simulink library "MQM_lib"  (Simulink 7.5)
settings: Solver=ode45  StartTime=0.0  StopTime=10.0  RelTol=1e-3
values from neighbouring files (symbols this model uses):
  pMQM_Nm_MaxPreloadTrq_C = Simulink.Parameter    [MQM_par.m]
  pMQM_Nm_ShfTqLowrCrossHiThd_C = Simulink.Parameter    [MQM_par.m]
  pMQM_Nm_ShfTqLowrCrossThd_C = Simulink.Parameter    [MQM_par.m]
  pMQM_Nm_ShfTqUpprCrossHiThd_C = Simulink.Parameter    [MQM_par.m]
  pMQM_Nm_ShfTqUpprCrossThd_C = Simulink.Parameter    [MQM_par.m]
  pMQM_Nm_TqRecoverThd_C = Simulink.Parameter    [MQM_par.m]
  pMQM_r_ShfNearZeroFilterFac_C = Simulink.Parameter    [MQM_par.m]
  pMQM_r_ShfPastZeroFilterFac_C = Simulink.Parameter    [MQM_par.m]
  pMQM_r_ShfZeroCrsFilterFac_C = Simulink.Parameter    [MQM_par.m]
  pMQM_s_ShfTqZeroCrossTiout_C = Simulink.Parameter    [MQM_par.m]
undefined symbols (not defined in the file or in its folder): p_single_Minus_M, p_single_Plus_M, p_single_Zero_M
libraries: BaseOperationLib_Browser x48, simulink x1
settings Model: Creator=wuaibin  LastModifiedBy=wuaibin

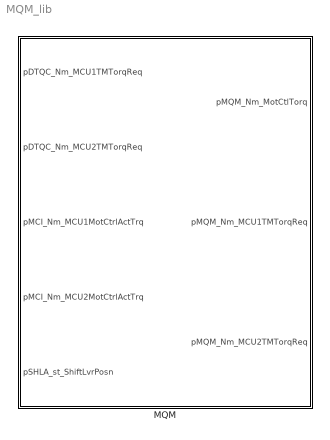
== system MQM_lib ==
  MQM : Subsystem  TreatAsAtomicUnit=on

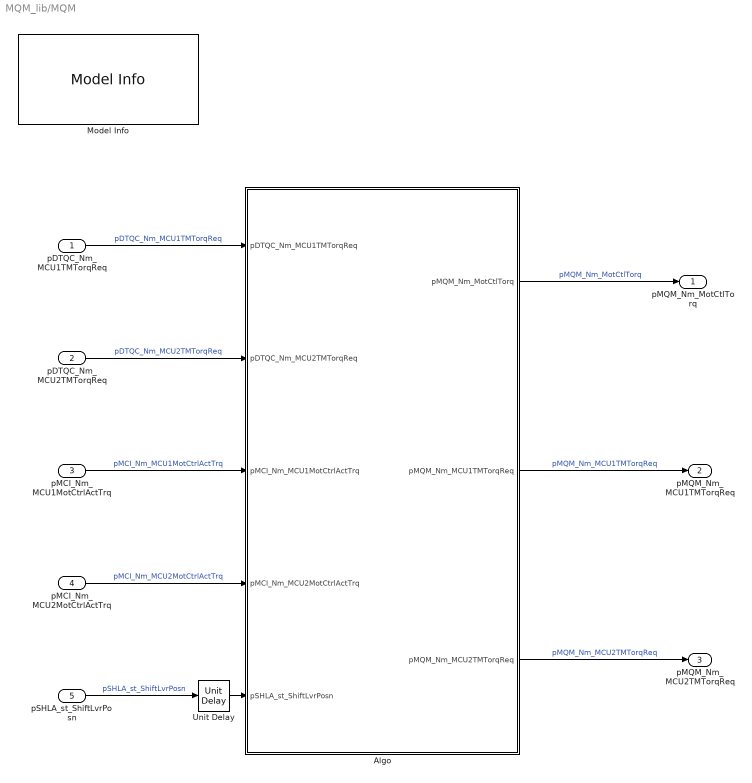
== system MQM_lib/MQM ==
  pDTQC_Nm_MCU1TMTorqReq : Inport
  pDTQC_Nm_MCU2TMTorqReq : Inport  Port=2
  pMCI_Nm_MCU1MotCtrlActTrq : Inport  Port=3
  pMCI_Nm_MCU2MotCtrlActTrq : Inport  Port=4
  pSHLA_st_ShiftLvrPosn : Inport  Port=5
  Algo : Subsystem
  Model Info : simulink/Model-Wide Utilities/Model Info  SystemSampleTime=-1  InitialBlockCM=None  BlockCM=None  Frame=on  DisplayStringWithTags=Model Info\nCreated: %<Created>\nCreator: %<Creator>  HorizontalTextAlignment=Center  LeftAlignmentValue=0.5  SourceBlockDiagram=untitled  TagMaxNumber=20
  Unit Delay : BaseOperationLib_Browser/Discrete Unchanged /Unit Delay  X0=0  SampleTime=-1
  pMQM_Nm_MotCtlTorq : Outport  OutDataType=fixdt(1, 16)  OutScaling=2^0
  pMQM_Nm_MCU1TMTorqReq : Outport  Port=2
  pMQM_Nm_MCU2TMTorqReq : Outport  Port=3
  wires:
  Unit Delay/1 -> Algo/5(pSHLA_st_ShiftLvrPosn)
  pDTQC_Nm_MCU1TMTorqReq/1 -> Algo/1(pDTQC_Nm_MCU1TMTorqReq)  "pDTQC_Nm_MCU1TMTorqReq"
  pDTQC_Nm_MCU2TMTorqReq/1 -> Algo/2(pDTQC_Nm_MCU2TMTorqReq)  "pDTQC_Nm_MCU2TMTorqReq"
  Algo/3(pMQM_Nm_MCU2TMTorqReq) -> pMQM_Nm_MCU2TMTorqReq/1  "pMQM_Nm_MCU2TMTorqReq"
  Algo/2(pMQM_Nm_MCU1TMTorqReq) -> pMQM_Nm_MCU1TMTorqReq/1  "pMQM_Nm_MCU1TMTorqReq"
  Algo/1(pMQM_Nm_MotCtlTorq) -> pMQM_Nm_MotCtlTorq/1  "pMQM_Nm_MotCtlTorq"
  pMCI_Nm_MCU1MotCtrlActTrq/1 -> Algo/3(pMCI_Nm_MCU1MotCtrlActTrq)  "pMCI_Nm_MCU1MotCtrlActTrq"
  pMCI_Nm_MCU2MotCtrlActTrq/1 -> Algo/4(pMCI_Nm_MCU2MotCtrlActTrq)  "pMCI_Nm_MCU2MotCtrlActTrq"
  pSHLA_st_ShiftLvrPosn/1 -> Unit Delay/1  "pSHLA_st_ShiftLvrPosn"

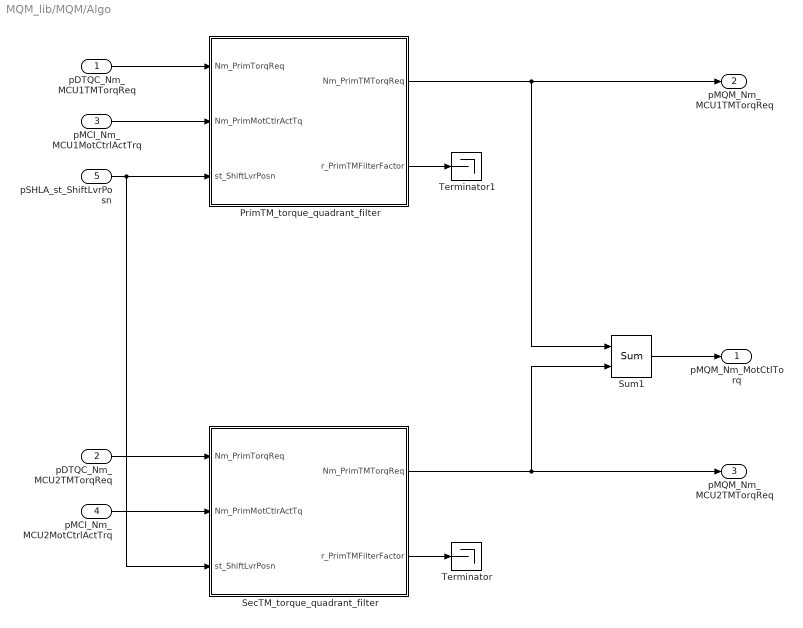
== system MQM_lib/MQM/Algo ==
  pDTQC_Nm_MCU1TMTorqReq : Inport
  pDTQC_Nm_MCU2TMTorqReq : Inport  Port=2
  pMCI_Nm_MCU1MotCtrlActTrq : Inport  Port=3
  pMCI_Nm_MCU2MotCtrlActTrq : Inport  Port=4
  pSHLA_st_ShiftLvrPosn : Inport  Port=5
  PrimTM_torque_quadrant_filter : Subsystem
  SecTM_torque_quadrant_filter : Subsystem
  Sum1 : BaseOperationLib_Browser/Math Operations Changed/Sum  Inputs=++  InputSameDT=on  OutMin=[]  OutMax=[]  OutDataType=fixdt(1, 16)  OutScaling=2^0  SaturateOnIntegerOverflow=on
  Terminator : Terminator
  Terminator1 : Terminator
  pMQM_Nm_MotCtlTorq : Outport  OutDataType=fixdt(1, 16)  OutScaling=2^0
  pMQM_Nm_MCU1TMTorqReq : Outport  Port=2
  pMQM_Nm_MCU2TMTorqReq : Outport  Port=3
  wires:
  pDTQC_Nm_MCU1TMTorqReq/1 -> PrimTM_torque_quadrant_filter/1(Nm_PrimTorqReq)
  pDTQC_Nm_MCU2TMTorqReq/1 -> SecTM_torque_quadrant_filter/1(Nm_PrimTorqReq)
  pMCI_Nm_MCU1MotCtrlActTrq/1 -> PrimTM_torque_quadrant_filter/2(Nm_PrimMotCtlrActTq)
  pSHLA_st_ShiftLvrPosn/1 -> SecTM_torque_quadrant_filter/3(st_ShiftLvrPosn), PrimTM_torque_quadrant_filter/3(st_ShiftLvrPosn)
  pMCI_Nm_MCU2MotCtrlActTrq/1 -> SecTM_torque_quadrant_filter/2(Nm_PrimMotCtlrActTq)
  SecTM_torque_quadrant_filter/2(r_PrimTMFilterFactor) -> Terminator/1
  PrimTM_torque_quadrant_filter/2(r_PrimTMFilterFactor) -> Terminator1/1
  PrimTM_torque_quadrant_filter/1(Nm_PrimTMTorqReq) -> pMQM_Nm_MCU1TMTorqReq/1, Sum1/1
  SecTM_torque_quadrant_filter/1(Nm_PrimTMTorqReq) -> pMQM_Nm_MCU2TMTorqReq/1, Sum1/2
  Sum1/1 -> pMQM_Nm_MotCtlTorq/1

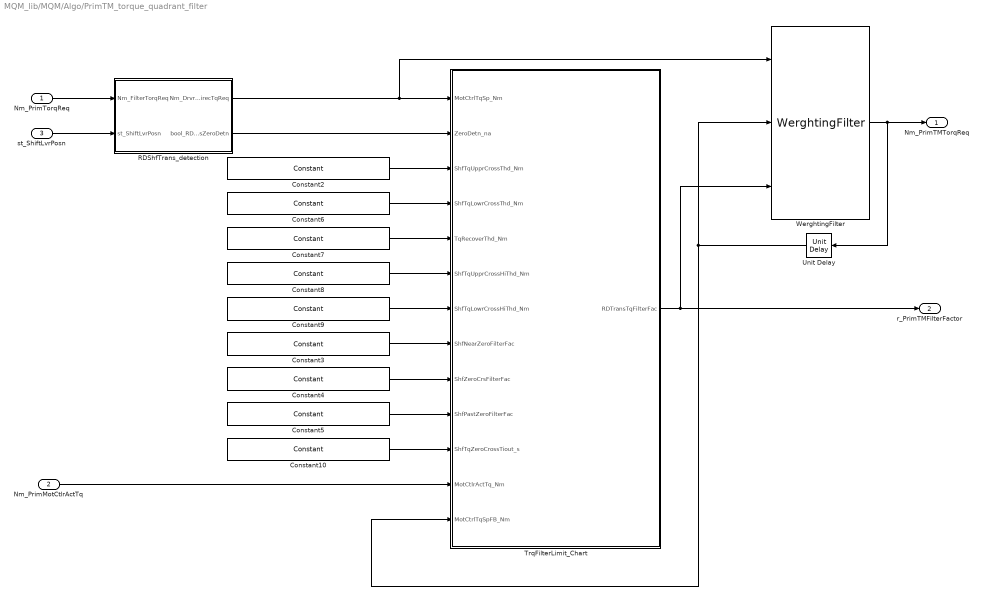
== system MQM_lib/MQM/Algo/PrimTM_torque_quadrant_filter ==
  Nm_PrimTorqReq : Inport
  Nm_PrimMotCtlrActTq : Inport  Port=2
  st_ShiftLvrPosn : Inport  Port=3
  Constant10 : BaseOperationLib_Browser/Sources&Sinks/Constant  Value=pMQM_s_ShfTqZeroCrossTiout_C  OutMin=[]  OutMax=[]  OutDataType=fixdt(1, 16)  ConRadixGroup=Use specified scaling  OutScaling=2^0  OutDataTypeStr=Inherit: Inherit from 'Constant value'
  Constant2 : BaseOperationLib_Browser/Sources&Sinks/Constant  Value=pMQM_Nm_ShfTqUpprCrossThd_C  OutMin=[]  OutMax=[]  OutDataType=fixdt(1, 16)  ConRadixGroup=Use specified scaling  OutScaling=2^0  OutDataTypeStr=Inherit: Inherit from 'Constant value'
  Constant3 : BaseOperationLib_Browser/Sources&Sinks/Constant  Value=pMQM_r_ShfNearZeroFilterFac_C  OutMin=[]  OutMax=[]  OutDataType=fixdt(1, 16)  ConRadixGroup=Use specified scaling  OutScaling=2^0  OutDataTypeStr=Inherit: Inherit from 'Constant value'
  Constant4 : BaseOperationLib_Browser/Sources&Sinks/Constant  Value=pMQM_r_ShfZeroCrsFilterFac_C  OutMin=[]  OutMax=[]  OutDataType=fixdt(1, 16)  ConRadixGroup=Use specified scaling  OutScaling=2^0  OutDataTypeStr=Inherit: Inherit from 'Constant value'
  Constant5 : BaseOperationLib_Browser/Sources&Sinks/Constant  Value=pMQM_r_ShfPastZeroFilterFac_C  OutMin=[]  OutMax=[]  OutDataType=fixdt(1, 16)  ConRadixGroup=Use specified scaling  OutScaling=2^0  OutDataTypeStr=Inherit: Inherit from 'Constant value'
  Constant6 : BaseOperationLib_Browser/Sources&Sinks/Constant  Value=pMQM_Nm_ShfTqLowrCrossThd_C  OutMin=[]  OutMax=[]  OutDataType=fixdt(1, 16)  ConRadixGroup=Use specified scaling  OutScaling=2^0  OutDataTypeStr=Inherit: Inherit from 'Constant value'
  Constant7 : BaseOperationLib_Browser/Sources&Sinks/Constant  Value=pMQM_Nm_TqRecoverThd_C  OutMin=[]  OutMax=[]  OutDataType=fixdt(1, 16)  ConRadixGroup=Use specified scaling  OutScaling=2^0  OutDataTypeStr=Inherit: Inherit from 'Constant value'
  Constant8 : BaseOperationLib_Browser/Sources&Sinks/Constant  Value=pMQM_Nm_ShfTqUpprCrossHiThd_C  OutMin=[]  OutMax=[]  OutDataType=fixdt(1, 16)  ConRadixGroup=Use specified scaling  OutScaling=2^0  OutDataTypeStr=Inherit: Inherit from 'Constant value'
  Constant9 : BaseOperationLib_Browser/Sources&Sinks/Constant  Value=pMQM_Nm_ShfTqLowrCrossHiThd_C  OutMin=[]  OutMax=[]  OutDataType=fixdt(1, 16)  ConRadixGroup=Use specified scaling  OutScaling=2^0  OutDataTypeStr=Inherit: Inherit from 'Constant value'
  RDShfTrans_detection : Subsystem
  TrqFilterLimit_Chart : Stateflow chart  TreatAsAtomicUnit=on
  Unit Delay : BaseOperationLib_Browser/Discrete Unchanged /Unit Delay  X0=0  SampleTime=-1
  WerghtingFilter : BaseOperationLib_Browser/Discontinuities Unchanged/WerghtingFilter  SystemSampleTime=-1
  Nm_PrimTMTorqReq : Outport
  r_PrimTMFilterFactor : Outport  Port=2
  wires:
  Constant10/1 -> TrqFilterLimit_Chart/11(ShfTqZeroCrossTiout_s)
  RDShfTrans_detection/1(Nm_DrvrDirecTqReq) -> WerghtingFilter/1, TrqFilterLimit_Chart/1(MotCtrlTqSp_Nm)
  Constant9/1 -> TrqFilterLimit_Chart/7(ShfTqLowrCrossHiThd_Nm)
  Constant8/1 -> TrqFilterLimit_Chart/6(ShfTqUpprCrossHiThd_Nm)
  Constant7/1 -> TrqFilterLimit_Chart/5(TqRecoverThd_Nm)
  Constant6/1 -> TrqFilterLimit_Chart/4(ShfTqLowrCrossThd_Nm)
  Constant2/1 -> TrqFilterLimit_Chart/3(ShfTqUpprCrossThd_Nm)
  st_ShiftLvrPosn/1 -> RDShfTrans_detection/2(st_ShiftLvrPosn)
  Constant5/1 -> TrqFilterLimit_Chart/10(ShfPastZeroFilterFac)
  Constant4/1 -> TrqFilterLimit_Chart/9(ShfZeroCrsFilterFac)
  Constant3/1 -> TrqFilterLimit_Chart/8(ShfNearZeroFilterFac)
  Nm_PrimMotCtlrActTq/1 -> TrqFilterLimit_Chart/12(MotCtlrActTq_Nm)
  Nm_PrimTorqReq/1 -> RDShfTrans_detection/1(Nm_FilterTorqReq)
  WerghtingFilter/1 -> Nm_PrimTMTorqReq/1, Unit Delay/1
  Unit Delay/1 -> TrqFilterLimit_Chart/13(MotCtrlTqSpFB_Nm), WerghtingFilter/2
  TrqFilterLimit_Chart/1(RDTransTqFilterFac) -> r_PrimTMFilterFactor/1, WerghtingFilter/3
  RDShfTrans_detection/2(bool_RDTransZeroDetn) -> TrqFilterLimit_Chart/2(ZeroDetn_na)

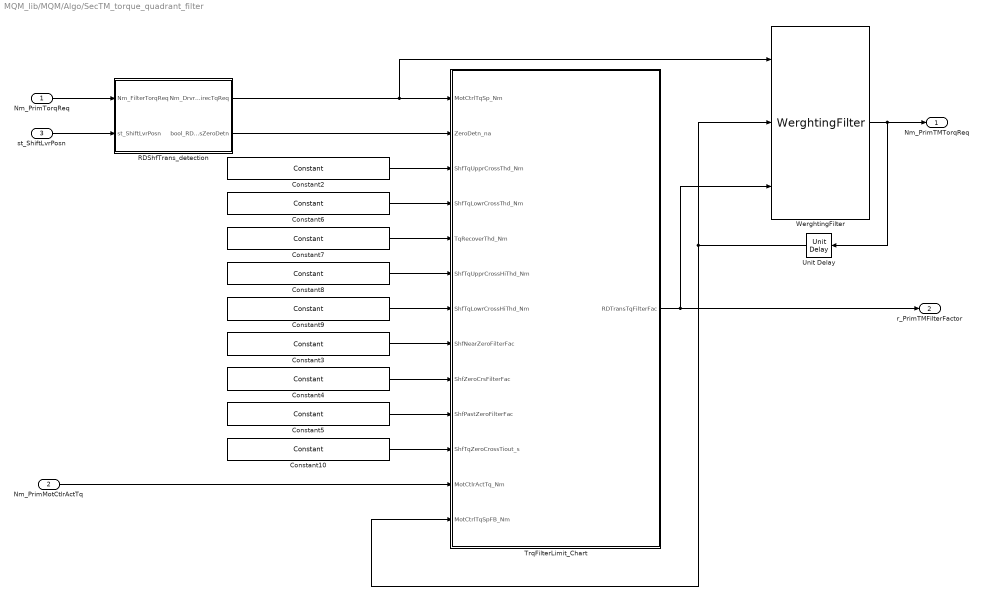
== system MQM_lib/MQM/Algo/SecTM_torque_quadrant_filter ==
  Nm_PrimTorqReq : Inport
  Nm_PrimMotCtlrActTq : Inport  Port=2
  st_ShiftLvrPosn : Inport  Port=3
  Constant10 : BaseOperationLib_Browser/Sources&Sinks/Constant  Value=pMQM_s_ShfTqZeroCrossTiout_C  OutMin=[]  OutMax=[]  OutDataType=fixdt(1, 16)  ConRadixGroup=Use specified scaling  OutScaling=2^0  OutDataTypeStr=Inherit: Inherit from 'Constant value'
  Constant2 : BaseOperationLib_Browser/Sources&Sinks/Constant  Value=pMQM_Nm_ShfTqUpprCrossThd_C  OutMin=[]  OutMax=[]  OutDataType=fixdt(1, 16)  ConRadixGroup=Use specified scaling  OutScaling=2^0  OutDataTypeStr=Inherit: Inherit from 'Constant value'
  Constant3 : BaseOperationLib_Browser/Sources&Sinks/Constant  Value=pMQM_r_ShfNearZeroFilterFac_C  OutMin=[]  OutMax=[]  OutDataType=fixdt(1, 16)  ConRadixGroup=Use specified scaling  OutScaling=2^0  OutDataTypeStr=Inherit: Inherit from 'Constant value'
  Constant4 : BaseOperationLib_Browser/Sources&Sinks/Constant  Value=pMQM_r_ShfZeroCrsFilterFac_C  OutMin=[]  OutMax=[]  OutDataType=fixdt(1, 16)  ConRadixGroup=Use specified scaling  OutScaling=2^0  OutDataTypeStr=Inherit: Inherit from 'Constant value'
  Constant5 : BaseOperationLib_Browser/Sources&Sinks/Constant  Value=pMQM_r_ShfPastZeroFilterFac_C  OutMin=[]  OutMax=[]  OutDataType=fixdt(1, 16)  ConRadixGroup=Use specified scaling  OutScaling=2^0  OutDataTypeStr=Inherit: Inherit from 'Constant value'
  Constant6 : BaseOperationLib_Browser/Sources&Sinks/Constant  Value=pMQM_Nm_ShfTqLowrCrossThd_C  OutMin=[]  OutMax=[]  OutDataType=fixdt(1, 16)  ConRadixGroup=Use specified scaling  OutScaling=2^0  OutDataTypeStr=Inherit: Inherit from 'Constant value'
  Constant7 : BaseOperationLib_Browser/Sources&Sinks/Constant  Value=pMQM_Nm_TqRecoverThd_C  OutMin=[]  OutMax=[]  OutDataType=fixdt(1, 16)  ConRadixGroup=Use specified scaling  OutScaling=2^0  OutDataTypeStr=Inherit: Inherit from 'Constant value'
  Constant8 : BaseOperationLib_Browser/Sources&Sinks/Constant  Value=pMQM_Nm_ShfTqUpprCrossHiThd_C  OutMin=[]  OutMax=[]  OutDataType=fixdt(1, 16)  ConRadixGroup=Use specified scaling  OutScaling=2^0  OutDataTypeStr=Inherit: Inherit from 'Constant value'
  Constant9 : BaseOperationLib_Browser/Sources&Sinks/Constant  Value=pMQM_Nm_ShfTqLowrCrossHiThd_C  OutMin=[]  OutMax=[]  OutDataType=fixdt(1, 16)  ConRadixGroup=Use specified scaling  OutScaling=2^0  OutDataTypeStr=Inherit: Inherit from 'Constant value'
  RDShfTrans_detection : Subsystem
  TrqFilterLimit_Chart : Stateflow chart  TreatAsAtomicUnit=on
  Unit Delay : BaseOperationLib_Browser/Discrete Unchanged /Unit Delay  X0=0  SampleTime=-1
  WerghtingFilter : BaseOperationLib_Browser/Discontinuities Unchanged/WerghtingFilter  SystemSampleTime=-1
  Nm_PrimTMTorqReq : Outport
  r_PrimTMFilterFactor : Outport  Port=2
  wires:
  RDShfTrans_detection/2(bool_RDTransZeroDetn) -> TrqFilterLimit_Chart/2(ZeroDetn_na)
  TrqFilterLimit_Chart/1(RDTransTqFilterFac) -> WerghtingFilter/3, r_PrimTMFilterFactor/1
  Unit Delay/1 -> WerghtingFilter/2, TrqFilterLimit_Chart/13(MotCtrlTqSpFB_Nm)
  WerghtingFilter/1 -> Unit Delay/1, Nm_PrimTMTorqReq/1
  Nm_PrimTorqReq/1 -> RDShfTrans_detection/1(Nm_FilterTorqReq)
  Nm_PrimMotCtlrActTq/1 -> TrqFilterLimit_Chart/12(MotCtlrActTq_Nm)
  Constant3/1 -> TrqFilterLimit_Chart/8(ShfNearZeroFilterFac)
  Constant4/1 -> TrqFilterLimit_Chart/9(ShfZeroCrsFilterFac)
  Constant5/1 -> TrqFilterLimit_Chart/10(ShfPastZeroFilterFac)
  st_ShiftLvrPosn/1 -> RDShfTrans_detection/2(st_ShiftLvrPosn)
  Constant2/1 -> TrqFilterLimit_Chart/3(ShfTqUpprCrossThd_Nm)
  Constant6/1 -> TrqFilterLimit_Chart/4(ShfTqLowrCrossThd_Nm)
  Constant7/1 -> TrqFilterLimit_Chart/5(TqRecoverThd_Nm)
  Constant8/1 -> TrqFilterLimit_Chart/6(ShfTqUpprCrossHiThd_Nm)
  Constant9/1 -> TrqFilterLimit_Chart/7(ShfTqLowrCrossHiThd_Nm)
  RDShfTrans_detection/1(Nm_DrvrDirecTqReq) -> TrqFilterLimit_Chart/1(MotCtrlTqSp_Nm), WerghtingFilter/1
  Constant10/1 -> TrqFilterLimit_Chart/11(ShfTqZeroCrossTiout_s)

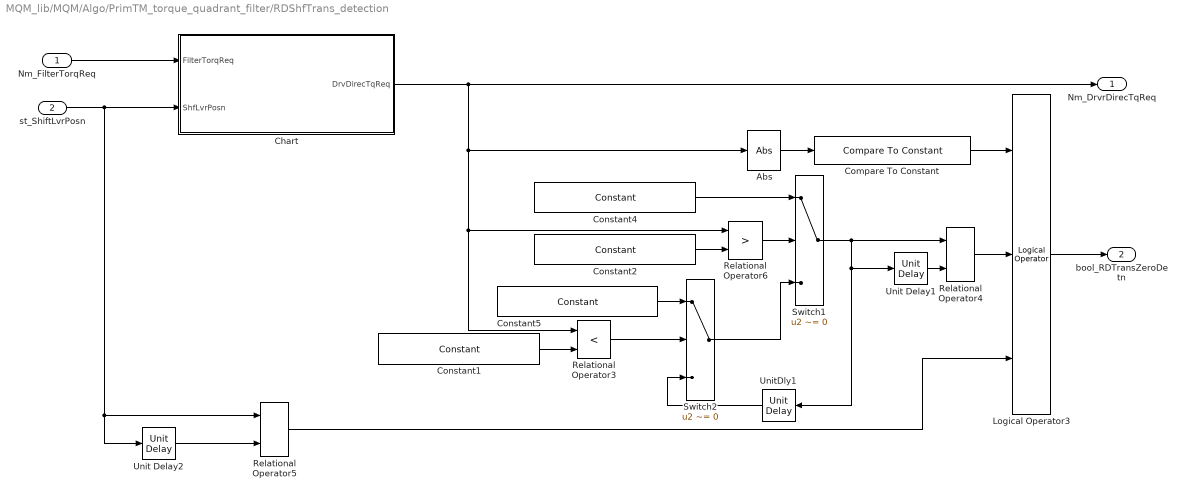
== system MQM_lib/MQM/Algo/PrimTM_torque_quadrant_filter/RDShfTrans_detection ==
  Nm_FilterTorqReq : Inport
  st_ShiftLvrPosn : Inport  Port=2
  Abs : BaseOperationLib_Browser/Math Operations Changed/Abs  OutMax=[]  OutDataType=fixdt(1, 16)  OutScaling=2^0  SaturateOnIntegerOverflow=on
  Chart : Stateflow chart  TreatAsAtomicUnit=on
  Compare To Constant : BaseOperationLib_Browser/Logic Operations Changed/Compare To Constant  SystemSampleTime=-1  relop=>=  const=pMQM_Nm_MaxPreloadTrq_C
  Constant1 : BaseOperationLib_Browser/Sources&Sinks/Constant  Value=p_single_Zero_M  OutMin=[]  OutMax=[]  OutDataType=fixdt(1, 16)  ConRadixGroup=Use specified scaling  OutScaling=2^0  OutDataTypeStr=Inherit: Inherit from 'Constant value'
  Constant2 : BaseOperationLib_Browser/Sources&Sinks/Constant  Value=p_single_Zero_M  OutMin=[]  OutMax=[]  OutDataType=fixdt(1, 16)  ConRadixGroup=Use specified scaling  OutScaling=2^0  OutDataTypeStr=Inherit: Inherit from 'Constant value'
  Constant4 : BaseOperationLib_Browser/Sources&Sinks/Constant  Value=p_single_Plus_M  OutMin=[]  OutMax=[]  OutDataType=fixdt(1, 16)  ConRadixGroup=Use specified scaling  OutScaling=2^0  OutDataTypeStr=Inherit: Inherit from 'Constant value'
  Constant5 : BaseOperationLib_Browser/Sources&Sinks/Constant  Value=p_single_Minus_M  OutMin=[]  OutMax=[]  OutDataType=fixdt(1, 16)  ConRadixGroup=Use specified scaling  OutScaling=2^0  OutDataTypeStr=Inherit: Inherit from 'Constant value'
  Logical Operator3 : BaseOperationLib_Browser/Logic Operations Changed/Logical Operator  Operator=AND  Inputs=3  AllPortsSameDT=off  OutDataTypeMode=boolean  LogicDataType=PDT_Bool  OutDataTypeStr=boolean
  Relational Operator3 : RelationalOperator  Operator=<  LogicOutDataTypeMode=Specify via dialog  LogicDataType=PDT_Bool  OutDataTypeStr=PDT_Bool  InputSameDT=on
      mask Display: patch([0 1 1 1 .75], [1 1 0 .75 1], [0 1 0]);
  Relational Operator4 : BaseOperationLib_Browser/Logic Operations Changed/Relational Operator  Operator=~=  InputSameDT=on  LogicOutDataTypeMode=Specify via dialog  LogicDataType=PDT_Bool  OutDataTypeStr=PDT_Bool
  Relational Operator5 : BaseOperationLib_Browser/Logic Operations Changed/Relational Operator  Operator=~=  InputSameDT=on  LogicOutDataTypeMode=Specify via dialog  LogicDataType=PDT_Bool  OutDataTypeStr=PDT_Bool
  Relational Operator6 : RelationalOperator  Operator=>  LogicOutDataTypeMode=Specify via dialog  LogicDataType=PDT_Bool  OutDataTypeStr=PDT_Bool  InputSameDT=on
      mask Display: patch([0 1 1 1 .75], [1 1 0 .75 1], [0 1 0]);
  Switch1 : Switch  Criteria=u2 ~= 0  Threshold=1  SaturateOnIntegerOverflow=on  InputSameDT=on
      mask Display: patch([0 1 1 1 .75], [1 1 0 .75 1], [0 1 0]);
  Switch2 : Switch  Criteria=u2 ~= 0  Threshold=1  SaturateOnIntegerOverflow=on  InputSameDT=on
      mask Display: patch([0 1 1 1 .75], [1 1 0 .75 1], [0 1 0]);
  Unit Delay1 : BaseOperationLib_Browser/Discrete Unchanged /Unit Delay  X0=0  SampleTime=-1
  Unit Delay2 : BaseOperationLib_Browser/Discrete Unchanged /Unit Delay  X0=0  SampleTime=-1
  UnitDly1 : BaseOperationLib_Browser/Discrete Unchanged /Unit Delay  X0=0  SampleTime=-1
  Nm_DrvrDirecTqReq : Outport
  bool_RDTransZeroDetn : Outport  Port=2
  wires:
  Relational Operator5/1 -> Logical Operator3/3
  Unit Delay2/1 -> Relational Operator5/2
  Constant5/1 -> Switch2/1
  Constant1/1 -> Relational Operator3/2
  Constant4/1 -> Switch1/1
  UnitDly1/1 -> Switch2/3
  Switch2/1 -> Switch1/3
  Relational Operator3/1 -> Switch2/2
  Switch1/1 -> Unit Delay1/1, UnitDly1/1, Relational Operator4/1
  Relational Operator6/1 -> Switch1/2
  Constant2/1 -> Relational Operator6/2
  st_ShiftLvrPosn/1 -> Unit Delay2/1, Relational Operator5/1, Chart/2(ShfLvrPosn)
  Nm_FilterTorqReq/1 -> Chart/1(FilterTorqReq)
  Chart/1(DrvDirecTqReq) -> Abs/1, Relational Operator3/1, Relational Operator6/1, Nm_DrvrDirecTqReq/1
  Logical Operator3/1 -> bool_RDTransZeroDetn/1
  Compare To Constant/1 -> Logical Operator3/1
  Abs/1 -> Compare To Constant/1
  Unit Delay1/1 -> Relational Operator4/2
  Relational Operator4/1 -> Logical Operator3/2

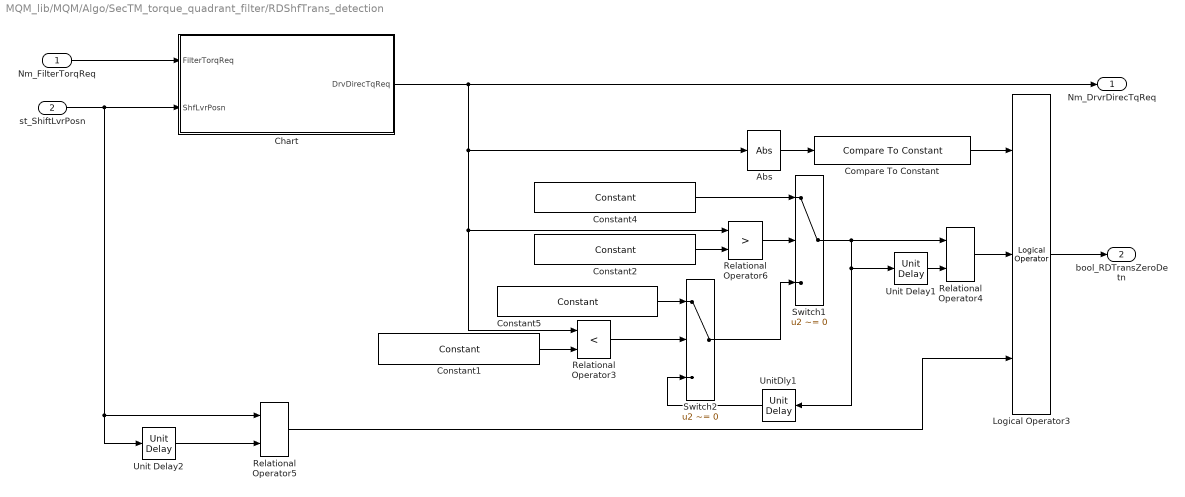
== system MQM_lib/MQM/Algo/SecTM_torque_quadrant_filter/RDShfTrans_detection ==
  Nm_FilterTorqReq : Inport
  st_ShiftLvrPosn : Inport  Port=2
  Abs : BaseOperationLib_Browser/Math Operations Changed/Abs  OutMax=[]  OutDataType=fixdt(1, 16)  OutScaling=2^0  SaturateOnIntegerOverflow=on
  Chart : Stateflow chart  TreatAsAtomicUnit=on
  Compare To Constant : BaseOperationLib_Browser/Logic Operations Changed/Compare To Constant  SystemSampleTime=-1  relop=>=  const=pMQM_Nm_MaxPreloadTrq_C
  Constant1 : BaseOperationLib_Browser/Sources&Sinks/Constant  Value=p_single_Zero_M  OutMin=[]  OutMax=[]  OutDataType=fixdt(1, 16)  ConRadixGroup=Use specified scaling  OutScaling=2^0  OutDataTypeStr=Inherit: Inherit from 'Constant value'
  Constant2 : BaseOperationLib_Browser/Sources&Sinks/Constant  Value=p_single_Zero_M  OutMin=[]  OutMax=[]  OutDataType=fixdt(1, 16)  ConRadixGroup=Use specified scaling  OutScaling=2^0  OutDataTypeStr=Inherit: Inherit from 'Constant value'
  Constant4 : BaseOperationLib_Browser/Sources&Sinks/Constant  Value=p_single_Plus_M  OutMin=[]  OutMax=[]  OutDataType=fixdt(1, 16)  ConRadixGroup=Use specified scaling  OutScaling=2^0  OutDataTypeStr=Inherit: Inherit from 'Constant value'
  Constant5 : BaseOperationLib_Browser/Sources&Sinks/Constant  Value=p_single_Minus_M  OutMin=[]  OutMax=[]  OutDataType=fixdt(1, 16)  ConRadixGroup=Use specified scaling  OutScaling=2^0  OutDataTypeStr=Inherit: Inherit from 'Constant value'
  Logical Operator3 : BaseOperationLib_Browser/Logic Operations Changed/Logical Operator  Operator=AND  Inputs=3  AllPortsSameDT=off  OutDataTypeMode=boolean  LogicDataType=PDT_Bool  OutDataTypeStr=boolean
  Relational Operator3 : RelationalOperator  Operator=<  LogicOutDataTypeMode=Specify via dialog  LogicDataType=PDT_Bool  OutDataTypeStr=PDT_Bool  InputSameDT=on
      mask Display: patch([0 1 1 1 .75], [1 1 0 .75 1], [0 1 0]);
  Relational Operator4 : BaseOperationLib_Browser/Logic Operations Changed/Relational Operator  Operator=~=  InputSameDT=on  LogicOutDataTypeMode=Specify via dialog  LogicDataType=PDT_Bool  OutDataTypeStr=PDT_Bool
  Relational Operator5 : BaseOperationLib_Browser/Logic Operations Changed/Relational Operator  Operator=~=  InputSameDT=on  LogicOutDataTypeMode=Specify via dialog  LogicDataType=PDT_Bool  OutDataTypeStr=PDT_Bool
  Relational Operator6 : RelationalOperator  Operator=>  LogicOutDataTypeMode=Specify via dialog  LogicDataType=PDT_Bool  OutDataTypeStr=PDT_Bool  InputSameDT=on
      mask Display: patch([0 1 1 1 .75], [1 1 0 .75 1], [0 1 0]);
  Switch1 : Switch  Criteria=u2 ~= 0  Threshold=1  SaturateOnIntegerOverflow=on  InputSameDT=on
      mask Display: patch([0 1 1 1 .75], [1 1 0 .75 1], [0 1 0]);
  Switch2 : Switch  Criteria=u2 ~= 0  Threshold=1  SaturateOnIntegerOverflow=on  InputSameDT=on
      mask Display: patch([0 1 1 1 .75], [1 1 0 .75 1], [0 1 0]);
  Unit Delay1 : BaseOperationLib_Browser/Discrete Unchanged /Unit Delay  X0=0  SampleTime=-1
  Unit Delay2 : BaseOperationLib_Browser/Discrete Unchanged /Unit Delay  X0=0  SampleTime=-1
  UnitDly1 : BaseOperationLib_Browser/Discrete Unchanged /Unit Delay  X0=0  SampleTime=-1
  Nm_DrvrDirecTqReq : Outport
  bool_RDTransZeroDetn : Outport  Port=2
  wires:
  Relational Operator4/1 -> Logical Operator3/2
  Unit Delay1/1 -> Relational Operator4/2
  Abs/1 -> Compare To Constant/1
  Compare To Constant/1 -> Logical Operator3/1
  Logical Operator3/1 -> bool_RDTransZeroDetn/1
  Chart/1(DrvDirecTqReq) -> Nm_DrvrDirecTqReq/1, Relational Operator6/1, Relational Operator3/1, Abs/1
  Nm_FilterTorqReq/1 -> Chart/1(FilterTorqReq)
  st_ShiftLvrPosn/1 -> Chart/2(ShfLvrPosn), Relational Operator5/1, Unit Delay2/1
  Constant2/1 -> Relational Operator6/2
  Relational Operator6/1 -> Switch1/2
  Switch1/1 -> Relational Operator4/1, UnitDly1/1, Unit Delay1/1
  Relational Operator3/1 -> Switch2/2
  Switch2/1 -> Switch1/3
  UnitDly1/1 -> Switch2/3
  Constant4/1 -> Switch1/1
  Constant1/1 -> Relational Operator3/2
  Constant5/1 -> Switch2/1
  Unit Delay2/1 -> Relational Operator5/2
  Relational Operator5/1 -> Logical Operator3/3

== stateflow chart MQM/Algo/SecTM_torque_quadrant_filter/RDShfTrans_detection/Chart ==
  state TQ_D
    en:
    DrvDirecTqReq=FilterTorqReq;
    du:
    DrvDirecTqReq=FilterTorqReq;
  state TQ_R
    en:
    DrvDirecTqReq=-FilterTorqReq;
    du:
    DrvDirecTqReq=-FilterTorqReq;
  TQ_D -> TQ_R : [ShfLvrPosn==ShiftLvrPosnTyp.SHL_R]
  TQ_R -> TQ_D : [ShfLvrPosn==ShiftLvrPosnTyp.SHL_D]
  (default) -> TQ_D
  data: FilterTorqReq input single; ShfLvrPosn input uint8; DrvDirecTqReq output single

== stateflow chart MQM/Algo/SecTM_torque_quadrant_filter/TrqFilterLimit_Chart ==
  state TorqueNoFilter
    en:
    RDTransTqFilterFac = 1;
    RisingZeroDetn_na=false;
    FallingZeroDetn_na=false;
    du:
    RDTransTqFilterFac = 1;
  state Shifting
    state ShiftZeroCrossingFilter
      en:
      RDTransTqFilterFac = ShfZeroCrsFilterFac;
      du:
      RDTransTqFilterFac = ShfZeroCrsFilterFac;
    state ShiftNearZeroFilter
      en:
      RDTransTqFilterFac = ShfNearZeroFilterFac;
      du:
      RDTransTqFilterFac = ShfNearZeroFilterFac;
    state ShiftPastZeroFilter
      en:
      RDTransTqFilterFac = ShfPastZeroFilterFac;
      du:
      RDTransTqFilterFac = ShfPastZeroFilterFac;
    ShiftNearZeroFilter -> ShiftZeroCrossingFilter : [(RisingZeroDetn_na&&MotCtlrActTq_Nm>= ShfTqUpprCrossThd_Nm)|| ...
        | (FallingZeroDetn_na&&MotCtlrActTq_Nm<=ShfTqLowrCrossThd_Nm)]
    ShiftZeroCrossingFilter -> ShiftPastZeroFilter : [(RisingZeroDetn_na&&MotCtlrActTq_Nm>= ShfTqUpprCrossHiThd_Nm)|| ...
        | (FallingZeroDetn_na&&MotCtlrActTq_Nm<=ShfTqLowrCrossHiThd_Nm)]
    (default) -> ShiftNearZeroFilter
  (default) -> TorqueNoFilter
  TorqueNoFilter -> Shifting [order 1] : [ZeroDetn_na&&(MotCtrlTqSp_Nm<0)]
      | {RisingZeroDetn_na=false;
      | FallingZeroDetn_na=true;}
  TorqueNoFilter -> Shifting [order 2] : [ZeroDetn_na&&(MotCtrlTqSp_Nm>0)]
      | {RisingZeroDetn_na=true;
      | FallingZeroDetn_na=false;}
  Shifting -> TorqueNoFilter : [(abs(MotCtrlTqSp_Nm-MotCtrlTqSpFB_Nm)<=TqRecoverThd_Nm)|| ...
      | (after(ShfTqZeroCrossTiout_s,sec))]
  data: MotCtrlTqSp_Nm input double; ZeroDetn_na input double; FallingZeroDetn_na local boolean; RDTransTqFilterFac output single; ShfTqUpprCrossThd_Nm input double; ShfTqLowrCrossThd_Nm input double; TqRecoverThd_Nm input double; ShfTqUpprCrossHiThd_Nm input double; ShfTqLowrCrossHiThd_Nm input double; ShfNearZeroFilterFac input double; ShfZeroCrsFilterFac input double; ShfPastZeroFilterFac input double; ShfTqZeroCrossTiout_s input double; MotCtlrActTq_Nm input double; MotCtrlTqSpFB_Nm input double; RisingZeroDetn_na local boolean

== stateflow chart MQM/Algo/PrimTM_torque_quadrant_filter/RDShfTrans_detection/Chart ==
  state TQ_D
    en:
    DrvDirecTqReq=FilterTorqReq;
    du:
    DrvDirecTqReq=FilterTorqReq;
  state TQ_R
    en:
    DrvDirecTqReq=-FilterTorqReq;
    du:
    DrvDirecTqReq=-FilterTorqReq;
  TQ_D -> TQ_R : [ShfLvrPosn==ShiftLvrPosnTyp.SHL_R]
  TQ_R -> TQ_D : [ShfLvrPosn==ShiftLvrPosnTyp.SHL_D]
  (default) -> TQ_D
  data: FilterTorqReq input single; ShfLvrPosn input uint8; DrvDirecTqReq output single

== stateflow chart MQM/Algo/PrimTM_torque_quadrant_filter/TrqFilterLimit_Chart ==
  state TorqueNoFilter
    en:
    RDTransTqFilterFac = 1;
    RisingZeroDetn_na=false;
    FallingZeroDetn_na=false;
    du:
    RDTransTqFilterFac = 1;
  state Shifting
    state ShiftZeroCrossingFilter
      en:
      RDTransTqFilterFac = ShfZeroCrsFilterFac;
      du:
      RDTransTqFilterFac = ShfZeroCrsFilterFac;
    state ShiftNearZeroFilter
      en:
      RDTransTqFilterFac = ShfNearZeroFilterFac;
      du:
      RDTransTqFilterFac = ShfNearZeroFilterFac;
    state ShiftPastZeroFilter
      en:
      RDTransTqFilterFac = ShfPastZeroFilterFac;
      du:
      RDTransTqFilterFac = ShfPastZeroFilterFac;
    ShiftNearZeroFilter -> ShiftZeroCrossingFilter : [(RisingZeroDetn_na&&MotCtlrActTq_Nm>= ShfTqUpprCrossThd_Nm)|| ...
        | (FallingZeroDetn_na&&MotCtlrActTq_Nm<=ShfTqLowrCrossThd_Nm)]
    ShiftZeroCrossingFilter -> ShiftPastZeroFilter : [(RisingZeroDetn_na&&MotCtlrActTq_Nm>= ShfTqUpprCrossHiThd_Nm)|| ...
        | (FallingZeroDetn_na&&MotCtlrActTq_Nm<=ShfTqLowrCrossHiThd_Nm)]
    (default) -> ShiftNearZeroFilter
  (default) -> TorqueNoFilter
  TorqueNoFilter -> Shifting [order 1] : [ZeroDetn_na&&(MotCtrlTqSp_Nm<0)]
      | {RisingZeroDetn_na=false;
      | FallingZeroDetn_na=true;}
  TorqueNoFilter -> Shifting [order 2] : [ZeroDetn_na&&(MotCtrlTqSp_Nm>0)]
      | {RisingZeroDetn_na=true;
      | FallingZeroDetn_na=false;}
  Shifting -> TorqueNoFilter : [(abs(MotCtrlTqSp_Nm-MotCtrlTqSpFB_Nm)<=TqRecoverThd_Nm)|| ...
      | (after(ShfTqZeroCrossTiout_s,sec))]
  data: MotCtrlTqSp_Nm input double; ZeroDetn_na input double; FallingZeroDetn_na local boolean; RDTransTqFilterFac output single; ShfTqUpprCrossThd_Nm input double; ShfTqLowrCrossThd_Nm input double; TqRecoverThd_Nm input double; ShfTqUpprCrossHiThd_Nm input double; ShfTqLowrCrossHiThd_Nm input double; ShfNearZeroFilterFac input double; ShfZeroCrsFilterFac input double; ShfPastZeroFilterFac input double; ShfTqZeroCrossTiout_s input double; MotCtlrActTq_Nm input double; MotCtrlTqSpFB_Nm input double; RisingZeroDetn_na local boolean
